simulink model "BLDC_180deg_hall_misalign_filtered"  (R2024a)
settings: Solver=ode15s  StartTime=0.0  StopTime=10  RelTol=1e-3
undefined symbols (not defined in the file or in its folder): HallError1, HallError2, HallError3, WrappedHallError1
libraries: simulink x7, slpidlib x1
settings Model: Creator=matthewhasman  LastModifiedBy=matthewhasman

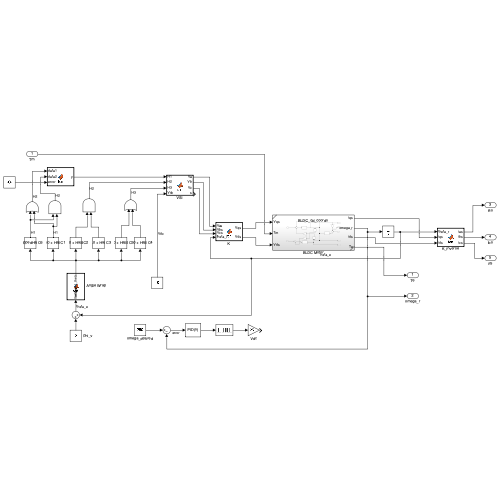
[thumbnail: Simulink's stored preview of the top-level diagram]
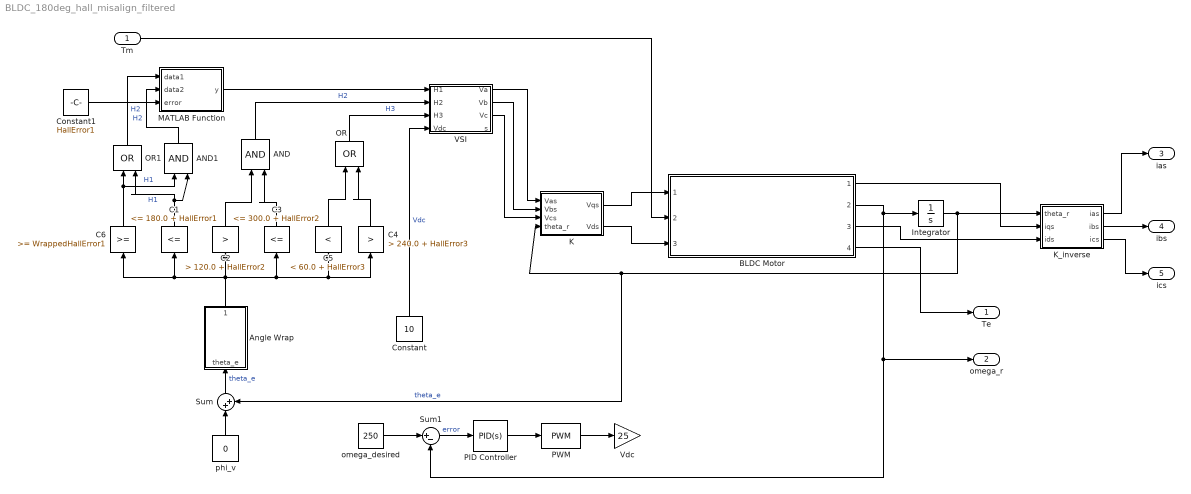
== system BLDC_180deg_hall_misalign_filtered ==
  Tm : Inport
  AND : Logic  IconShape=distinctive  AllPortsSameDT=off  OutDataTypeStr=boolean
  AND1 : Logic  IconShape=distinctive  AllPortsSameDT=off  OutDataTypeStr=boolean
  Angle Wrap : MATLAB Function  TreatAsAtomicUnit=on
  BLDC Motor : Subsystem  ReferencedSubsystem=BLDC_qd_coords
  C1 : simulink/Logic and Bit Operations/Compare To Constant  relop=<=  const=180.0 + HallError1  OutDataTypeStr=boolean
  C2 : simulink/Logic and Bit Operations/Compare To Constant  relop=>  const=120.0 + HallError2  OutDataTypeStr=boolean
  C3 : simulink/Logic and Bit Operations/Compare To Constant  relop=<=  const=300.0 + HallError2  OutDataTypeStr=boolean
  C4 : simulink/Logic and Bit Operations/Compare To Constant  relop=>  const=240.0 + HallError3  OutDataTypeStr=boolean
  C5 : simulink/Logic and Bit Operations/Compare To Constant  relop=<  const=60.0 + HallError3  OutDataTypeStr=boolean
  C6 : simulink/Logic and Bit Operations/Compare To Constant  relop=>=  const=WrappedHallError1  OutDataTypeStr=boolean
  Constant : Constant  Value=10
  Constant1 : Constant  Value=HallError1
  Integrator : Integrator
  K : MATLAB Function  TreatAsAtomicUnit=on
  K_inverse : MATLAB Function  TreatAsAtomicUnit=on
  MATLAB Function : MATLAB Function  TreatAsAtomicUnit=on
  OR : Logic  Operator=OR  IconShape=distinctive  AllPortsSameDT=off  OutDataTypeStr=boolean
  OR1 : Logic  Operator=OR  IconShape=distinctive  AllPortsSameDT=off  OutDataTypeStr=boolean
  PID Controller : slpidlib/PID Controller  Controller=PID  Form=Parallel  TimeDomain=Continuous-time  UseExternalTs=off  SampleTime=-1  IntegratorMethod=Forward Euler  FilterMethod=Forward Euler  ControllerParametersSource=internal  P=8  I=5  UseKiTs=off  D=1  UseExternalDerivativeSource=off  N=100  UseFilter=on  TunerSelectOption=Transfer Function Based (PID Tuner App)  InitialConditionSource=internal  InitialConditionForIntegrator=0  InitialConditionForFilter=0  DifferentiatorICPrevScaledInput=0  ExternalReset=none  TrackingMode=off  Kt=1  LimitOutput=off  SatLimitsSource=internal  UpperSaturationLimit=inf  LowerSaturationLimit=-inf  LinearizeAsGain=on  AntiWindupMode=none  Kb=1  LimitIntegrator=off  UpperIntegratorSaturationLimit=inf  LowerIntegratorSaturationLimit=-inf  POutMin=[]  POutMax=[]  IOutMin=[]  IOutMax=[]  DOutMin=[]  DOutMax=[]  NOutMin=[]  NOutMax=[]  SumOutMin=[]  SumOutMax=[]  SaturationOutMin=[]  SaturationOutMax=[]  PParamMin=[]  PParamMax=[]  IParamMin=[]  IParamMax=[]  DParamMin=[]  DParamMax=[]  NParamMin=[]  NParamMax=[]  KbParamMin=[]  KbParamMax=[]  KtParamMin=[]  KtParamMax=[]  KbOutMin=[]  KbOutMax=[]  KtOutMin=[]  KtOutMax=[]  IntegratorOutMin=[]  IntegratorOutMax=[]  FilterOutMin=[]  FilterOutMax=[]  SumI1OutMin=[]  SumI1OutMax=[]  SumI2OutMin=[]  SumI2OutMax=[]  SumI3OutMin=[]  SumI3OutMax=[]  SumI4OutMin=[]  SumI4OutMax=[]  SumDOutMin=[]  SumDOutMax=[]  DifferentiatorOutMin=[]  DifferentiatorOutMax=[]  FilterDiffOutCoefMin=[]  FilterDiffOutCoefMax=[]  ReciprocalOutMin=[]  ReciprocalOutMax=[]  SumDenOutMin=[]  SumDenOutMax=[]  SumNumOutMin=[]  SumNumOutMax=[]  DivideOutMin=[]  DivideOutMax=[]  UdiffTsProdOutMin=[]  UdiffTsProdOutMax=[]  NTsProdOutMin=[]  NTsProdOutMax=[]  UintegralTsProdOutMin=[]  UintegralTsProdOutMax=[]  UngainTsProdOutMin=[]  UngainTsProdOutMax=[]  ClampingZeroOutDataTypeStr=Inherit: Inherit via back propagation  ClampingZeroOutMin=[]  ClampingZeroOutMax=[]  FilterDenConstantOutDataTypeStr=Inherit: Inherit via back propagation  FilterDenConstantOutMin=[]  FilterDenConstantOutMax=[]  PCopyOutDataTypeStr=Inherit: Inherit via back propagation  PCopyOutMin=[]  PCopyOutMax=[]  NCopyOutDataTypeStr=Inherit: Inherit via back propagation  NCopyOutMin=[]  NCopyOutMax=[]  IntegratorContinuousStateAttributes=''  IntegratorStateMustResolveToSignalObject=off  IntegratorRTWStateStorageClass=Auto  FilterContinuousStateAttributes=''  FilterStateMustResolveToSignalObject=off  FilterRTWStateStorageClass=Auto  ParallelPVariant=InternalParameters  IdealPVariant=Disabled  IVariant=InternalParameters  DVariant=InternalParameters  IntegratorVariant=Continuous  SatVariant=Disabled  AWVariant=Passthrough  PCopyVariant=Disabled  TRVariant=Disabled  FdbkBlocksVariant=Forward  IdealPFdbkVariant=Disabled  SatFdbkVariant=Disabled  DerivativeFilterVariant=ContFilter  NVariant=InternalParameters  NCopyVariant=Disabled  FilterICVariant=InternalICsFilter  IntegratorICVariant=InternalICs  ExternalResetVariant=Disabled  TRSumVariant=Passthrough  SumFdbkVariant=Disabled  SumVariant=Sum_PID  TsampFilterVariant=InternalTs  TsampNgainVariant=Passthrough  TsampIntegralVariant=Disabled_SignalSpec  ExternalSaturationOutDataTypeStr=Inherit: Same as second input  DerivativeSourceVariant=ErrorSignal
  PWM : simulink/Discontinuities/PWM  DisableCoverage=on  Period=0.0001  InitialDelay=0  DisallowZeroDutyCycle=off  RunAtFixedTimeIntervals=off  SampleTime=0.1
  Sum : Sum  Inputs=|++
  Sum1 : Sum  Inputs=|+-
  VSI : MATLAB Function  TreatAsAtomicUnit=on
  Vdc : Gain  Gain=25
  omega_desired : Constant  Value=250
  phi_v : Constant  Value=0
  Te : Outport
  omega_r : Outport  Port=2
  ias : Outport  Port=3
  ibs : Outport  Port=4
  ics : Outport  Port=5
  wires:
  Integrator/1 -> K_inverse/1(theta_r), K/4(theta_r), Sum/2  "theta_e"
  BLDC Motor/1 -> K_inverse/2(iqs)
  BLDC Motor/3 -> K_inverse/3(ids)
  K/1(Vqs) -> BLDC Motor/1
  Tm/1 -> BLDC Motor/2
  phi_v/1 -> Sum/1
  VSI/1(Va) -> K/1(Vas)
  VSI/2(Vb) -> K/2(Vbs)
  VSI/3(Vc) -> K/3(Vcs)
  omega_desired/1 -> Sum1/1
  Sum1/1 -> PID Controller/1  "error"
  PID Controller/1 -> PWM/1
  PWM/1 -> Vdc/1
  Constant/1 -> VSI/4(Vdc)  "Vdc"
  K/2(Vds) -> BLDC Motor/3
  Sum/1 -> Angle Wrap/1(theta_e)  "theta_e"
  Angle Wrap/1(wrapped_theta) -> C2/1, C5/1, C4/1, C3/1, C6/1, C1/1
  C2/1 -> AND/1
  C3/1 -> AND/2
  AND/1 -> VSI/2(H2)  "H2"
  C5/1 -> OR/1
  C4/1 -> OR/2
  OR/1 -> VSI/3(H3)  "H3"
  BLDC Motor/2 -> omega_r/1, Sum1/2, Integrator/1
  BLDC Motor/4 -> Te/1
  K_inverse/1(ias) -> ias/1
  K_inverse/2(ibs) -> ibs/1
  K_inverse/3(ics) -> ics/1
  C6/1 -> AND1/1, OR1/1  "H1"
  C1/1 -> AND1/2, OR1/2  "H1"
  MATLAB Function/1(y) -> VSI/1(H1)
  OR1/1 -> MATLAB Function/1(data1)  "H2"
  AND1/1 -> MATLAB Function/2(data2)  "H2"
  Constant1/1 -> MATLAB Function/3(error)

== matlab function BLDC_180deg_hall_misalign_filtered/K ==
  data: Vas input; Vqs output; Vbs input; Vcs input; Vds output; theta_r input
function [Vqs, Vds] = fcn(Vas, Vbs, Vcs, theta_r)
offset = 2*pi/3;
k = (2/3)*[cos(theta_r), cos(theta_r - offset), cos(theta_r + offset);
           sin(theta_r), sin(theta_r - offset), sin(theta_r + offset)];

qds_voltage = k * [Vas; Vbs; Vcs];

Vqs = qds_voltage(1);
Vds = qds_voltage(2);

end

== matlab function BLDC_180deg_hall_misalign_filtered/K_inverse ==
  data: theta_r input; ias output; iqs input; ids input; ibs output; ics output
function [ias, ibs, ics] = fcn(theta_r, iqs, ids)
offset = 2*pi/3;
k_inverse = [cos(theta_r), sin(theta_r);
             cos(theta_r - offset), sin(theta_r - offset);
             cos(theta_r + offset), sin(theta_r + offset)];

abc_currents = k_inverse * [iqs; ids];

ias = abc_currents(1);
ibs = abc_currents(2);
ics = abc_currents(3);

end

== matlab function BLDC_180deg_hall_misalign_filtered/Angle Wrap ==
  data: theta_e input; wrapped_theta output
function wrapped_theta = fcn(theta_e)

wrapped_theta = wrapTo2Pi(theta_e) * 180 / pi;

== matlab function BLDC_180deg_hall_misalign_filtered/VSI ==
  data: Va output; H1 input; H2 input; H3 input; Vb output; Vc output; Vdc input; s output
function [Va, Vb, Vc, s] = fcn(H1, H2, H3, Vdc)

% Initialize T1, T2, T3
T1 = 0;
T2 = 0;
T3 = 0;
s=0;

% Determine T1, T2, T3 based on theta_e
if (H1 && H3)
    [T1, T2, T3] = deal(1, 0, 0);
    s=0;
elseif (H1 && ~H2 && ~H3)
    [T1, T2, T3] = deal(1, 1, 0);
    s=1;
elseif (H2 && H1)
    [T1, T2, T3] = deal(0, 1, 0);
    s=2;
elseif (H2 && ~H1 && ~H3)
    [T1, T2, T3] = deal(0, 1, 1);
    s=3;
elseif (H2 && H3)
    [T1, T2, T3] = deal(0, 0, 1);
    s=4;
else
    [T1, T2, T3] = deal(1, 0, 1);
    s=5;
end

% % Determine T1, T2, T3 based on theta_e
% if (H1 && H3)
%     [T1, T2, T3] = deal(1, 0, 1);
%     s=0;
% elseif (H1)
%     [T1, T2, T3] = deal(1, 0, 0);
%     s=1;
% elseif (H2 && H1)
%     [T1, T2, T3] = deal(1, 1, 0);
%     s=2;
% elseif (H2)
%     [T1, T2, T3] = deal(0, 1, 0);
%     s=3;
% elseif (H2 && H3)
%     [T1, T2, T3] = deal(0, 1, 1);
%     s=4;
% else
%     [T1, T2, T3] = deal(0, 0, 1);
%     s=5;
% end

% Matrix A for transformations
A = [2/3, -1/3, -1/3;
     -1/3, 2/3, -1/3;
     -1/3, -1/3, 2/3;];

% Create T vector
T = [T1; T2; T3];

% Compute Vabc
Vabc = Vdc * A * T;

Va = Vabc(1);
Vb = Vabc(2); 
Vc = Vabc(3); 

end

== matlab function BLDC_180deg_hall_misalign_filtered/MATLAB Function ==
  data: data1 input; y output; data2 input; error input
function y = fcn(data1, data2, error)

if error > 0
    y = data2;

else 
    y = data1;

end
